simulink model "case_1_lead_veh_sudden_stop"  (R2025b)
settings: Solver=VariableStepAuto  StartTime=0.0  StopTime=10.0  RelTol=1e-3
settings Model: Creator=admin  LastModifiedBy=admin

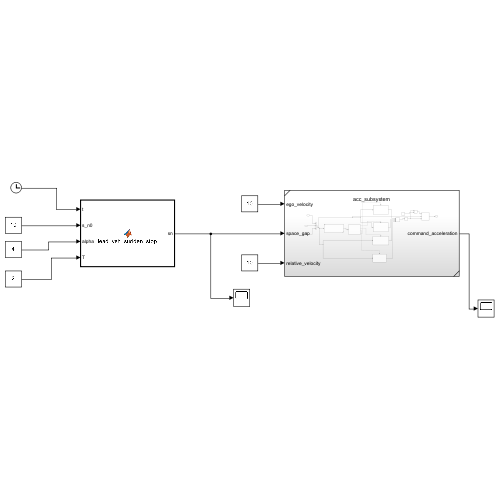
[thumbnail: Simulink's stored preview of the top-level diagram]
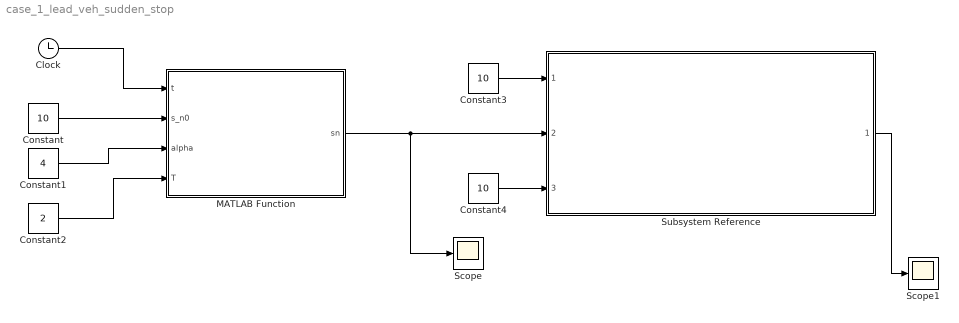
== system case_1_lead_veh_sudden_stop ==
  Clock : Clock
  Constant : Constant  Value=10
  Constant1 : Constant  Value=4
  Constant2 : Constant  Value=2
  Constant3 : Constant  Value=10
  Constant4 : Constant  Value=10
  MATLAB Function : MATLAB Function  TreatAsAtomicUnit=on
  Scope : Scope
      settings: ActiveDisplayYMinimum=-1.2499999999999998  ActiveDisplayYMaximum=11.25
  Scope1 : Scope
      settings: ActiveDisplayYMinimum=-1  ActiveDisplayYMaximum=1
  Subsystem Reference : Subsystem  ReferencedSubsystem=acc_subsystem
  wires:
  Clock/1 -> MATLAB Function/1(t)
  Constant/1 -> MATLAB Function/2(s_n0)
  Constant1/1 -> MATLAB Function/3(alpha)
  Constant2/1 -> MATLAB Function/4(T)
  Subsystem Reference/1 -> Scope1/1
  Constant3/1 -> Subsystem Reference/1
  Constant4/1 -> Subsystem Reference/3
  MATLAB Function/1(sn) -> Scope/1, Subsystem Reference/2

== matlab function case_1_lead_veh_sudden_stop/MATLAB Function ==
  data: t input; sn output; s_n0 input; alpha input; T input
function sn = lead_veh_sudden_stop(t, s_n0, alpha, T)
    if t < T
        sn = s_n0;
    else
        sn = max(-alpha * s_n0, 0);
    end
end
